simulink model "gtm_aeromodel"  (Simulink 7.2)
settings: Solver=ode45  StartTime=0.0  StopTime=10.0  RelTol=1e-3
undefined symbols (not defined in the file or in its folder): A_BLCG, A_BW, A_CW, A_FSCG, A_FSREF_in, A_SW, A_WLCG, A_WLREF, ALPHA0, bclowb, bclowbx_FMACH, bcmowb, bcmowbx_FHP, bcmowby_FMACH, cda, cdax_FLPDEF, cddr, cddrx_FMACH, cdo, cdox_FLPDEF, cdt1, cdt1x_mach, cdt2, cdt2x_mach, cdto, cdtox_mach, cdwb, cdwbx_FALPHA, cdwby_FMACH, clat, clatfr, clatfrx_FHP, clatfry_FMACH, clatx_mach, clawbfr, clawbfrx_FHP, clawbfry_FMACH, cldefr, cldefrx_FHP, cldefry_FMACH, cldtab, cldtabx_FMACH, clqwb, clqwbfr, clqwbfrx_FHP, clqwbfry_FMACH, clqwbx_mach, cltdd, cltddx_FHP, cltddy_FMACH, clwb, clwbtdd, clwbtddx_FHP, clwbtddy_FMACH, clwbx_FALPHA, clwby_FMACH, clwbzdd, clwbzddx_FHP, clwbzddy_FMACH, clzdd ... (+196)
libraries: model_lib x1
(part 1 of 10)
settings Model: Creator=E183308  LastModifiedBy=E183308

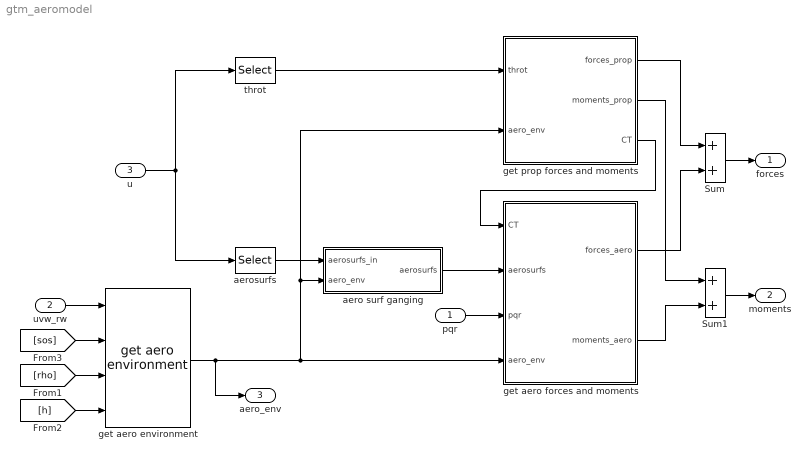
== system gtm_aeromodel ==
  pqr : Inport  OutDataType=sfix(16)  OutScaling=2^0
  uvw_rw : Inport  Port=2  OutDataType=sfix(16)  OutScaling=2^0
  u : Inport  Port=3  OutDataType=sfix(16)  OutScaling=2^0
  Sum : Sum  OutDataType=sfix(16)  OutScaling=2^0
  Sum1 : Sum  OutDataType=sfix(16)  OutScaling=2^0
  aero surf ganging : Subsystem
  aerosurfs : Selector  InputPortWidth=num_u  IndexOptions=Index vector (dialog)  Indices=vane_idx  OutputSizes=1
  get aero environment : model_lib/get aero environment  SystemSampleTime=-1
  get aero forces and moments : Subsystem
  get prop forces and moments : Subsystem
  throt : Selector  InputPortWidth=num_u  IndexOptions=Index vector (dialog)  Indices=throttle_idx  OutputSizes=1
  forces : Outport  OutDataType=sfix(16)  OutScaling=2^0
  moments : Outport  Port=2  OutDataType=sfix(16)  OutScaling=2^0
  aero_env : Outport  Port=3  OutDataType=sfix(16)  OutScaling=2^0
  wires:
  [h] -> get aero environment/4
  [sos] -> get aero environment/2
  [rho] -> get aero environment/3
  u/1 -> aerosurfs/1, throt/1
  uvw_rw/1 -> get aero environment/1
  throt/1 -> get prop forces and moments/1(throt)
  aerosurfs/1 -> aero surf ganging/1(aerosurfs_in)
  Sum/1 -> forces/1
  Sum1/1 -> moments/1
  get prop forces and moments/1(forces_prop) -> Sum/1
  get aero forces and moments/1(forces_aero) -> Sum/2
  get prop forces and moments/2(moments_prop) -> Sum1/1
  get prop forces and moments/3(CT) -> get aero forces and moments/1(CT)
  get aero forces and moments/2(moments_aero) -> Sum1/2
  pqr/1 -> get aero forces and moments/3(pqr)
  aero surf ganging/1(aerosurfs) -> get aero forces and moments/2(aerosurfs)
  get aero environment/1 -> get aero forces and moments/4(aero_env), aero surf ganging/2(aero_env), get prop forces and moments/2(aero_env), aero_env/1

== system gtm_aeromodel/aero surf ganging ==
  aerosurfs_in : Inport  OutDataType=sfix(16)  OutScaling=2^0
  aero_env : Inport  Port=2  OutDataType=sfix(16)  OutScaling=2^0
  Bus Creator : BusCreator  Inputs=13
  Bus Selector1 : BusSelector  OutputSignals=qbar
  Constant : Constant  Value=0  OutDataType=sfix(16)  OutScaling=2^0
  Constant1 : Constant  Value=0  OutDataType=sfix(16)  OutScaling=2^0
  Demux : Demux  Outputs=7
  FLAP/DSTAB : Lookup  InputValues=dstabx_FLPDEF  Table=dstab  OutDataType=sfix(16)  OutScaling=2^0  SaturateOnIntegerOverflow=on
  Gain : Gain  Gain=-1  ParameterDataType=sfix(16)  ParameterScaling=2^0  OutDataType=sfix(16)  OutScaling=2^0
  Gain{1..4} (4 alike) : Gain  ParameterDataType=sfix(16)  ParameterScaling=2^0  OutDataType=sfix(16)  OutScaling=2^0
  SPOILER : Subsystem
  aerosurfs : Outport  OutDataType=sfix(16)  OutScaling=2^0
  wires:
  Constant1/1 -> Bus Creator/6  "flgail"
  Constant/1 -> Bus Creator/8  "atab"
  Gain1/1 -> Bus Creator/11  "dsb"
  Gain4/1 -> Bus Creator/7  "ailr"
  Gain3/1 -> Bus Creator/13  "dsr"
  Gain2/1 -> Bus Creator/12  "dsl"
  Demux/5 -> SPOILER/3(splr)  "stab"
  SPOILER/3(dsr) -> Gain3/1  "dsr"
  SPOILER/2(dsl) -> Gain2/1  "dsl"
  SPOILER/1(dsb) -> Gain1/1  "dsb"
  Bus Selector1/1 -> SPOILER/2(Qdyn)
  aero_env/1 -> Bus Selector1/1
  FLAP/DSTAB/1 -> Bus Creator/5  "stab"
  Demux/6 -> FLAP/DSTAB/1, Bus Creator/9  "flap"
  Demux/1 -> SPOILER/1(halfdail), Gain4/1, Gain/1  "ail"
  Bus Creator/1 -> aerosurfs/1
  aerosurfs_in/1 -> Demux/1
  Demux/7 -> Bus Creator/10  "gear"
  Demux/4 -> Bus Creator/4  "eltab"
  Demux/3 -> Bus Creator/3  "rud"
  Gain/1 -> Bus Creator/2  "aill"
  Demux/2 -> Bus Creator/1  "elev"

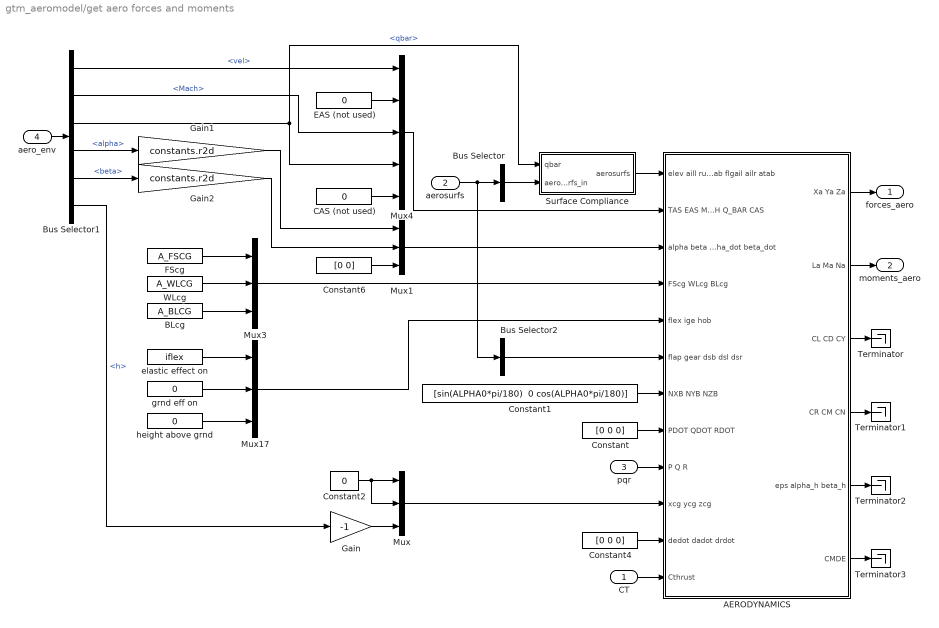
== system gtm_aeromodel/get aero forces and moments ==
  CT : Inport  OutDataType=sfix(16)  OutScaling=2^0
  aerosurfs : Inport  Port=2  OutDataType=sfix(16)  OutScaling=2^0
  pqr : Inport  Port=3  OutDataType=sfix(16)  OutScaling=2^0
  aero_env : Inport  Port=4  OutDataType=sfix(16)  OutScaling=2^0
  AERODYNAMICS : Subsystem
  BLcg : Constant  Value=A_BLCG  OutDataType=sfix(16)  OutScaling=2^0
  Bus Selector : BusSelector  OutputSignals=elev,aill,rud,eltab,stab,flgail,ailr,atab  OutputAsBus=on
  Bus Selector1 : BusSelector  OutputSignals=vel,Mach,qbar,alpha,beta,h
  Bus Selector2 : BusSelector  OutputSignals=flap,gear,dsb,dsl,dsr  OutputAsBus=on
  CAS (not used) : Constant  Value=0  OutDataType=sfix(16)  OutScaling=2^0
  Constant : Constant  Value=[0 0 0]  OutDataType=sfix(16)  OutScaling=2^0
  Constant1 : Constant  Value="[sin(ALPHA0*pi/180)  0 cos(ALPHA0*pi/180)]"  OutDataType=sfix(16)  OutScaling=2^0
  Constant2 : Constant  Value=0  OutDataType=sfix(16)  OutScaling=2^0
  Constant4 : Constant  Value=[0 0 0]  OutDataType=sfix(16)  OutScaling=2^0
  Constant6 : Constant  Value=[0 0]  OutDataType=sfix(16)  OutScaling=2^0
  EAS (not used) : Constant  Value=0  OutDataType=sfix(16)  OutScaling=2^0
  FScg : Constant  Value=A_FSCG  OutDataType=sfix(16)  OutScaling=2^0
  Gain : Gain  Gain=-1  ParameterDataType=sfix(16)  ParameterScaling=2^0  OutDataType=sfix(16)  OutScaling=2^0
  Gain1 : Gain  Gain=constants.r2d  ParameterDataType=sfix(16)  ParameterScaling=2^0  OutDataType=sfix(16)  OutScaling=2^0
  Gain2 : Gain  Gain=constants.r2d  ParameterDataType=sfix(16)  ParameterScaling=2^0  OutDataType=sfix(16)  OutScaling=2^0
  Mux : Mux  Inputs=3
  Mux1 : Mux  Inputs=[1 1 2]
  Mux17 : Mux  Inputs=3
  Mux3 : Mux  Inputs=3
  Mux4 : Mux  Inputs=5
  Surface Compliance : Subsystem
  Terminator{,1..3} (4 alike) : Terminator
  WLcg : Constant  Value=A_WLCG  OutDataType=sfix(16)  OutScaling=2^0
  elastic effect on : Constant  Value=iflex  OutDataType=sfix(16)  OutScaling=2^0
  grnd eff on : Constant  Value=0  OutDataType=sfix(16)  OutScaling=2^0
  height above grnd : Constant  Value=0  OutDataType=sfix(16)  OutScaling=2^0
  forces_aero : Outport  OutDataType=sfix(16)  OutScaling=2^0
  moments_aero : Outport  Port=2  OutDataType=sfix(16)  OutScaling=2^0
  wires:
  AERODYNAMICS/6(CMDE) -> Terminator3/1
  AERODYNAMICS/5(eps alpha_h beta_h) -> Terminator2/1
  AERODYNAMICS/4(CR CM CN) -> Terminator1/1
  AERODYNAMICS/3(CL CD CY) -> Terminator/1
  AERODYNAMICS/2(La Ma Na) -> moments_aero/1
  AERODYNAMICS/1("Xa Ya Za ") -> forces_aero/1
  Gain2/1 -> Mux1/2
  Gain1/1 -> Mux1/1
  Constant/1 -> AERODYNAMICS/8(PDOT QDOT RDOT)
  Constant1/1 -> AERODYNAMICS/7(NXB NYB NZB)
  pqr/1 -> AERODYNAMICS/9(P Q R)
  elastic effect on/1 -> Mux17/1
  grnd eff on/1 -> Mux17/2
  height above grnd/1 -> Mux17/3
  Bus Selector1/4 -> Gain1/1  "<alpha>"
  Mux1/1 -> AERODYNAMICS/3(alpha beta alpha_dot beta_dot)
  FScg/1 -> Mux3/1
  WLcg/1 -> Mux3/2
  BLcg/1 -> Mux3/3
  Mux3/1 -> AERODYNAMICS/4(FScg WLcg BLcg)
  Mux17/1 -> AERODYNAMICS/5(flex ige hob)
  EAS (not used)/1 -> Mux4/2
  Bus Selector1/3 -> Mux4/4, Surface Compliance/1(qbar)  "<qbar>"
  CAS (not used)/1 -> Mux4/5
  Bus Selector1/2 -> Mux4/3  "<Mach>"
  Mux4/1 -> AERODYNAMICS/2(TAS EAS MACH Q_BAR CAS)
  Constant6/1 -> Mux1/3
  Bus Selector1/5 -> Gain2/1  "<beta>"
  Bus Selector1/1 -> Mux4/1  "<vel>"
  aero_env/1 -> Bus Selector1/1
  Mux/1 -> AERODYNAMICS/10(xcg ycg zcg)
  Constant4/1 -> AERODYNAMICS/11(dedot dadot drdot)
  CT/1 -> AERODYNAMICS/12(Cthrust)
  Constant2/1 -> Mux/1, Mux/2
  Gain/1 -> Mux/3
  Bus Selector1/6 -> Gain/1  "<h>"
  aerosurfs/1 -> Bus Selector/1, Bus Selector2/1
  Bus Selector/1 -> Surface Compliance/2(aerosurfs_in)
  Bus Selector2/1 -> AERODYNAMICS/6(flap gear dsb dsl dsr)
  Surface Compliance/1(aerosurfs) -> AERODYNAMICS/1(elev aill rud eltab stab flgail ailr atab)

== system gtm_aeromodel/get prop forces and moments ==
  throt : Inport  OutDataType=sfix(16)  OutScaling=2^0
  aero_env : Inport  Port=2  OutDataType=sfix(16)  OutScaling=2^0
  Bus Selector : BusSelector  OutputSignals=qbar,Mach,h
  Constant1 : Constant  Value=4  VectorParams1D=off  OutDataType=sfix(16)  OutScaling=2^0
  Constant2 : Constant  Value=A_WLCG  VectorParams1D=off  OutDataType=sfix(16)  OutScaling=2^0
  ENGINE : Subsystem
  Engine inlet area (ft^2) : Constant  Value=12.57  VectorParams1D=off  OutDataType=sfix(16)  OutScaling=2^0
  Product3 : Product  Inputs=3  OutDataType=sfix(16)  OutScaling=2^0  RndMeth=Zero
  Terminator : Terminator
  Terminator1 : Terminator
  Terminator2 : Terminator
  forces_prop : Outport  OutDataType=sfix(16)  OutScaling=2^0
  moments_prop : Outport  Port=2  OutDataType=sfix(16)  OutScaling=2^0
  CT : Outport  Port=3  OutDataType=sfix(16)  OutScaling=2^0
  wires:
  throt/1 -> ENGINE/1(Thrust_Lever)
  ENGINE/1(Forces Prop) -> forces_prop/1
  ENGINE/2(Moments Prop) -> moments_prop/1
  ENGINE/3(CT) -> CT/1
  ENGINE/4(maxThrust) -> Terminator/1
  ENGINE/5(minThrust) -> Terminator1/1
  ENGINE/6(TRA) -> Terminator2/1
  Constant1/1 -> Product3/1
  Engine inlet area (ft^2)/1 -> Product3/2
  Product3/1 -> ENGINE/2(RamDrag0)
  Constant2/1 -> ENGINE/6(A_WLCG)
  aero_env/1 -> Bus Selector/1
  Bus Selector/1 -> Product3/3, ENGINE/3(Q_Bar0)  "<qbar>"
  Bus Selector/2 -> ENGINE/4(Mach)  "<Mach>"
  Bus Selector/3 -> ENGINE/5(Alt)  "<h>"

== system gtm_aeromodel/aero surf ganging/SPOILER ==
  note: isp
  halfdail : Inport  OutDataType=sfix(16)  OutScaling=2^0
  Qdyn : Inport  Port=2  OutDataType=sfix(16)  OutScaling=2^0
  splr : Inport  Port=3  OutDataType=sfix(16)  OutScaling=2^0
  Gain3 : Gain  Gain=-1  ParameterDataType=sfix(16)  ParameterScaling=2^0  OutDataType=sfix(16)  OutScaling=2^0  SaturateOnIntegerOverflow=on  OutDataTypeStr=Inherit: Same as input  ParamDataTypeStr=Inherit: Same as input
  Model Info : Subsystem  LoadFcn=slcm LoadBlock;  InitFcn=slcm('UpdateAllCMBlocksInThisModelInit')  mask(CMBlock){InitialSaveTempField=, InitialBlockCM=None, BlockCM=none, Frame=on, SaveTempField=, DisplayStringWithTags=|, MaskDisplayString=Model Name: SPOILER   Rev.: -\nDescription: Spoiler\nProgram: Planeview GV \nNext Block: ACTUATORS\nWritten by: G. Chan     Date: 06/28/00, HorizontalTextAlignment=Left, LeftAlignmentValue=0.02, SourceBlockDiagram=models, TagMaxNumber=20, CMTag1=, CMTag2=, CMTag3=, CMTag4=, CMTag5=, CMTag6=, CMTag7=, CMTag8=, CMTag9=, CMTag10=, CMTag11=, CMTag12=, CMTag13=, CMTag14=, CMTag15=, CMTag16=, CMTag17=, CMTag18=, CMTag19=, CMTag20=}
      mask DisplayStringWithTags=|
      | Model Name: SPOILER   Rev.: -
      | Description: Spoiler
      | Program: Planeview GV
      | Next Block: ACTUATORS
      | Written by: G. Chan     Date: 06/28/00
      mask help: This block allows revision control information to be displayed within the model.
      settings: CopyFcn=slcm CopyBlock;  DeleteFcn=slcm Cancel;  PostSaveFcn=slcm('UpdateAllCMBlocksInThisModel')  NameChangeFcn=slcm Rename;  OpenFcn=slcm
      mask Display: text(str2num(LeftAlignmentValue), 0.5, MaskDisplayString, 'HorizontalAlignment', HorizontalTextAlignment)
  Saturation : Saturate  UpperLimit=70  LowerLimit=0
  Saturation1 : Saturate  UpperLimit=70  LowerLimit=0
  Switch : Switch  Threshold=.5  SaturateOnIntegerOverflow=on  InputSameDT=on
  Switch1 : Switch  Threshold=.5  SaturateOnIntegerOverflow=on  InputSameDT=on
  dsl_ : Constant  Value=0  OutDataType=sfix(16)  OutScaling=2^0
  dsl_1 : Sum  OutDataType=sfix(16)  OutScaling=2^0  SaturateOnIntegerOverflow=on  InputSameDT=on  OutDataTypeStr=Inherit: Same as first input
  dslgear_1 : Subsystem  mask(2-D Table){y=dslgearx_FQ, z=dslgeary_DAILL, tab=dslgear}
      mask prompts: y "Y vector:"; z "Z vector:"; tab "Table:"
      mask help: 2-D Table Look Up. Enter monotonic Y and Z vectors and a matrix of 2-D tables. See the help for more info.
      mask Help: The Y and Z vectors must be monotonic.  Y  indexes into the columns of the 2-D table & Z indexes into the rows of the 2-D tables.   The input values are y and z respectively (e.g., top port = y).
      mask Display: plot(-10,-10,110,110,[90,50,10],[90,40,30],[90,50,10],[50,26,20],[90,50,10],[22,13,10])
  dsr_ : Constant  Value=0  OutDataType=sfix(16)  OutScaling=2^0
  dsr_1 : Sum  OutDataType=sfix(16)  OutScaling=2^0  SaturateOnIntegerOverflow=on  InputSameDT=on  OutDataTypeStr=Inherit: Same as first input
  dsrgear_ : Subsystem  mask(2-D Table){y=dsrgearx_FQ, z=dsrgeary_DAILR, tab=dsrgear}
      mask prompts: y "Y vector:"; z "Z vector:"; tab "Table:"
      mask help: 2-D Table Look Up. Enter monotonic Y and Z vectors and a matrix of 2-D tables. See the help for more info.
      mask Help: The Y and Z vectors must be monotonic.  Y  indexes into the columns of the 2-D table & Z indexes into the rows of the 2-D tables.   The input values are y and z respectively (e.g., top port = y).
      mask Display: plot(-10,-10,110,110,[90,50,10],[90,40,30],[90,50,10],[50,26,20],[90,50,10],[22,13,10])
  gearStatus3 : Constant  OutDataType=sfix(16)  OutScaling=2^0
  dsb : Outport  OutDataType=sfix(16)  OutScaling=2^0
  dsl : Outport  Port=2  OutDataType=sfix(16)  OutScaling=2^0
  dsr : Outport  Port=3  OutDataType=sfix(16)  OutScaling=2^0
  wires:
  halfdail/1 -> dsrgear_/2(Z), Gain3/1
  Qdyn/1 -> dslgear_1/1(Y), dsrgear_/1(Y)
  Gain3/1 -> dslgear_1/2(Z)
  dslgear_1/1(Interp Value) -> Switch/1
  dsrgear_/1(Interp Value) -> Switch1/1
  Saturation1/1 -> dsr/1
  dsr_1/1 -> Saturation1/1
  Saturation/1 -> dsl/1
  dsl_1/1 -> Saturation/1
  dsr_/1 -> Switch1/3
  dsl_/1 -> Switch/3
  Switch1/1 -> dsr_1/2
  gearStatus3/1 -> Switch1/2, Switch/2
  Switch/1 -> dsl_1/2
  splr/1 -> dsr_1/1, dsl_1/1, dsb/1

== system gtm_aeromodel/get aero forces and moments/AERODYNAMICS ==
  elev aill rud eltab stab flgail ailr atab : Inport  OutDataType=sfix(16)  OutScaling=2^0
  TAS EAS MACH Q_BAR CAS : Inport  Port=2  OutDataType=sfix(16)  OutScaling=2^0
  alpha beta alpha_dot beta_dot : Inport  Port=3  OutDataType=sfix(16)  OutScaling=2^0
  FScg WLcg BLcg : Inport  Port=4  OutDataType=sfix(16)  OutScaling=2^0
  flex ige hob : Inport  Port=5  OutDataType=sfix(16)  OutScaling=2^0
  flap gear dsb dsl dsr : Inport  Port=6  OutDataType=sfix(16)  OutScaling=2^0
  NXB NYB NZB : Inport  Port=7  OutDataType=sfix(16)  OutScaling=2^0
  PDOT QDOT RDOT : Inport  Port=8  OutDataType=sfix(16)  OutScaling=2^0
  P Q R : Inport  Port=9  OutDataType=sfix(16)  OutScaling=2^0
  xcg ycg zcg : Inport  Port=10  OutDataType=sfix(16)  OutScaling=2^0
  dedot dadot drdot : Inport  Port=11  OutDataType=sfix(16)  OutScaling=2^0
  Cthrust : Inport  Port=12  OutDataType=sfix(16)  OutScaling=2^0
  Aero Incidence Angles : Subsystem
  Force  Coefficients : Subsystem
  Moment Coefficients : Subsystem
  Mux : Mux  Inputs=3
  NONDIMRATE : Subsystem
  XFORMATION of  AERO FORCES and MOMENTS   to cg centered body axis : Subsystem
  sin2 : Fcn  Expr=-u[3]
  "Xa Ya Za " : Outport  OutDataType=sfix(16)  OutScaling=2^0  InitialOutput=0
  La Ma Na : Outport  Port=2  OutDataType=sfix(16)  OutScaling=2^0  InitialOutput=0
  CL CD CY : Outport  Port=3  OutDataType=sfix(16)  OutScaling=2^0  InitialOutput=0
  CR CM CN : Outport  Port=4  OutDataType=sfix(16)  OutScaling=2^0  InitialOutput=0
  eps alpha_h beta_h : Outport  Port=5  OutDataType=sfix(16)  OutScaling=2^0  InitialOutput=0
  CMDE : Outport  Port=6  OutDataType=sfix(16)  OutScaling=2^0  InitialOutput=0
  wires:
  Moment Coefficients/2(CMDE) -> CMDE/1
  NXB NYB NZB/1 -> Aero Incidence Angles/6(NXB NYB NZB), Moment Coefficients/9(NXB NYB NZB), Force  Coefficients/10(NXB NYB NZB)
  sin2/1 -> Aero Incidence Angles/2(alt), Moment Coefficients/7(alt), Force  Coefficients/8(alt)
  xcg ycg zcg/1 -> sin2/1
  Mux/1 -> eps alpha_h beta_h/1
  Aero Incidence Angles/3(betat) -> Mux/3, Force  Coefficients/12(beta_h), Moment Coefficients/12(beta_h)
  Aero Incidence Angles/1(eps) -> Mux/1, Force  Coefficients/2(eps)
  Aero Incidence Angles/2(alphat) -> Mux/2, Force  Coefficients/6(alpha_h), Moment Coefficients/5(alpha_h)
  Cthrust/1 -> Aero Incidence Angles/7(cthrust)
  PDOT QDOT RDOT/1 -> Force  Coefficients/11(PDOT QDOT RDOT), Moment Coefficients/10(PDOT QDOT RDOT)
  alpha beta alpha_dot beta_dot/1 -> Aero Incidence Angles/9(alpha beta alpha_dot beta_dot), NONDIMRATE/2(alpha beta eps_h alpha_h), Force  Coefficients/3(alpha beta alpha_dot beta_dot), Moment Coefficients/2(alpha beta alpha_dot beta_dot), XFORMATION of  AERO FORCES and MOMENTS   to cg centered body axis/3(alpha beta alpha_dot beta_dot)
  P Q R/1 -> Aero Incidence Angles/8(P Q R), NONDIMRATE/1(P Q R)
  TAS EAS MACH Q_BAR CAS/1 -> XFORMATION of  AERO FORCES and MOMENTS   to cg centered body axis/1(Vtas EASkts Mach Qdyn CASkts), Aero Incidence Angles/1(TAS EAS MACH Q_BAR CAS), NONDIMRATE/3(Vtas EASkts Mach Qdyn CASkts), Force  Coefficients/4(TAS EAS MACH Q_BAR CAS), Moment Coefficients/3(TAS EAS MACH Q_BAR CAS)
  XFORMATION of  AERO FORCES and MOMENTS   to cg centered body axis/2(La Ma Na) -> La Ma Na/1
  XFORMATION of  AERO FORCES and MOMENTS   to cg centered body axis/1(Xa Ya Za) -> "Xa Ya Za "/1
  dedot dadot drdot/1 -> Moment Coefficients/11(dedot dadot drdot)
  FScg WLcg BLcg/1 -> XFORMATION of  AERO FORCES and MOMENTS   to cg centered body axis/5(FScg WLcg BLcg)
  NONDIMRATE/1(P' Q' R') -> Force  Coefficients/5(P' Q' R'), Moment Coefficients/4(PHAT QHAT RHAT)
  flex ige hob/1 -> Aero Incidence Angles/3(flex ige hob), Moment Coefficients/1(flex ige hob), Force  Coefficients/1("flex ige hob ")
  elev aill rud eltab stab flgail ailr atab/1 -> Aero Incidence Angles/5(ctrl_surfaces), Moment Coefficients/6(elev aill rud eltab stab flgail ailr atab), Force  Coefficients/7(elev aill rud eltab stab flgail ailr atab)
  flap gear dsb dsl dsr/1 -> Aero Incidence Angles/4(flap gear dsb dsl dsr), Moment Coefficients/8(flap gear dsb dsl dsr), Force  Coefficients/9(flap gear dsb dsl dsr)
  Force  Coefficients/1(CL CD CY) -> XFORMATION of  AERO FORCES and MOMENTS   to cg centered body axis/2(CL CD CY), CL CD CY/1
  Moment Coefficients/1(CR CM CN) -> XFORMATION of  AERO FORCES and MOMENTS   to cg centered body axis/4(CR CM CN), CR CM CN/1

== system gtm_aeromodel/get aero forces and moments/Surface Compliance ==
  qbar : Inport  OutDataType=sfix(16)  OutScaling=2^0
  aerosurfs_in : Inport  Port=2  OutDataType=sfix(16)  OutScaling=2^0
  Aileron Compliance : Lookup  InputValues="[0  92  221]"  Table="[1  0.85  0.8]"  OutDataType=sfix(16)  OutScaling=2^0  SaturateOnIntegerOverflow=on
  Demux : Demux  Outputs=[1 1 6]
  Elevator Compliance : Lookup  InputValues=[0 46 132 200 300 400]  Table="[1   1  0.7  0.65 0.6 0.4]"  OutDataType=sfix(16)  OutScaling=2^0  SaturateOnIntegerOverflow=on
  Mux : Mux  Inputs=3
  Product : Product  OutDataType=sfix(16)  OutScaling=2^0  RndMeth=Zero
  Product1 : Product  OutDataType=sfix(16)  OutScaling=2^0  RndMeth=Zero
  aerosurfs : Outport  OutDataType=sfix(16)  OutScaling=2^0
  wires:
  Mux/1 -> aerosurfs/1
  Demux/1 -> Product/2
  Demux/2 -> Product1/2
  Product/1 -> Mux/1
  aerosurfs_in/1 -> Demux/1
  Demux/3 -> Mux/3
  Elevator Compliance/1 -> Product/1
  qbar/1 -> Aileron Compliance/1, Elevator Compliance/1
  Product1/1 -> Mux/2
  Aileron Compliance/1 -> Product1/1

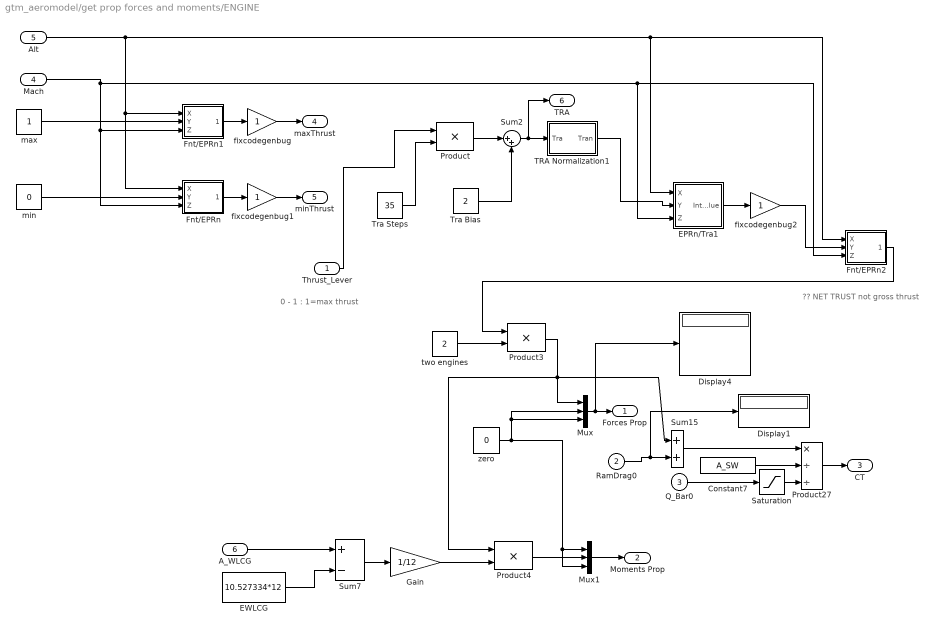
== system gtm_aeromodel/get prop forces and moments/ENGINE ==
  note: ?? NET TRUST not gross thrust
  note: 0 - 1 : 1=max thrust
  Thrust_Lever : Inport  OutDataType=sfix(16)  OutScaling=2^0
  RamDrag0 : Inport  Port=2  OutDataType=sfix(16)  OutScaling=2^0
  Q_Bar0 : Inport  Port=3  OutDataType=sfix(16)  OutScaling=2^0
  Mach : Inport  Port=4  OutDataType=sfix(16)  OutScaling=2^0
  Alt : Inport  Port=5  OutDataType=sfix(16)  OutScaling=2^0
  A_WLCG : Inport  Port=6  OutDataType=sfix(16)  OutScaling=2^0
  Constant7 : Constant  Value=A_SW  OutDataType=sfix(16)  OutScaling=2^0
  Display1 : Display
  Display4 : Display
  EPRn/Tra1 : Subsystem  mask(1-2-3 Table){@1=altvec, @2=sstravec, @3=machvec, @4=eprn_tra}
      mask prompts: @1 "X vector:"; @2 "Y vector:"; @3 "Z vector:"; @4 "Table:"
      mask help: 3-D Table Look Up. Enter monotonic X, Y and Z vectors and a matrix of 2-D tables. See the help for more info.
      mask init:
      | x=@1;y=@2;z=@3;tab=@4;
      mask Help: The X, Y and Z vectors must be monotonic.   The 3-D table is a horizontal concatenation of  2-D tables.  X  indexes into the columns of the 2-D tables & Y indexes into the rows of the 2-D tables.  Z indexes into the table levels (starting with the 1st 2-D table).   The input values are x, y and z respectively (e.g., top port = x).
      mask Display: plot([0 2 2 0 0],[0 0 2 2 0],[0 2 2.9 0.95 0],[2 2 2.7 2.7 2],[2 2.9 2.9 2 2],[0 0.85 2.7 2 0])
  EWLCG : Constant  Value=10.527334*12  OutDataType=sfix(16)  OutScaling=2^0
  Fnt/EPRn : Subsystem  mask(1-2-3 Table){@1=altvec, @2=sseprvec, @3=machvec, @4=fn_epr}
      mask prompts: @1 "X vector:"; @2 "Y vector:"; @3 "Z vector:"; @4 "Table:"
      mask help: 3-D Table Look Up. Enter monotonic X, Y and Z vectors and a matrix of 2-D tables. See the help for more info.
      mask init:
      | x=@1;y=@2;z=@3;tab=@4;
      mask Help: The X, Y and Z vectors must be monotonic.   The 3-D table is a horizontal concatenation of  2-D tables.  X  indexes into the columns of the 2-D tables & Y indexes into the rows of the 2-D tables.  Z indexes into the table levels (starting with the 1st 2-D table).   The input values are x, y and z respectively (e.g., top port = x).
      mask Display: plot([0 2 2 0 0],[0 0 2 2 0],[0 2 2.9 0.95 0],[2 2 2.7 2.7 2],[2 2.9 2.9 2 2],[0 0.85 2.7 2 0])
  Fnt/EPRn1 : Subsystem  mask(1-2-3 Table){@1=altvec, @2=sseprvec, @3=machvec, @4=fn_epr}
      mask prompts: @1 "X vector:"; @2 "Y vector:"; @3 "Z vector:"; @4 "Table:"
      mask help: 3-D Table Look Up. Enter monotonic X, Y and Z vectors and a matrix of 2-D tables. See the help for more info.
      mask init:
      | x=@1;y=@2;z=@3;tab=@4;
      mask Help: The X, Y and Z vectors must be monotonic.   The 3-D table is a horizontal concatenation of  2-D tables.  X  indexes into the columns of the 2-D tables & Y indexes into the rows of the 2-D tables.  Z indexes into the table levels (starting with the 1st 2-D table).   The input values are x, y and z respectively (e.g., top port = x).
      mask Display: plot([0 2 2 0 0],[0 0 2 2 0],[0 2 2.9 0.95 0],[2 2 2.7 2.7 2],[2 2.9 2.9 2 2],[0 0.85 2.7 2 0])
  Fnt/EPRn2 : Subsystem  mask(1-2-3 Table){@1=altvec, @2=sseprvec, @3=machvec, @4=fn_epr}
      mask prompts: @1 "X vector:"; @2 "Y vector:"; @3 "Z vector:"; @4 "Table:"
      mask help: 3-D Table Look Up. Enter monotonic X, Y and Z vectors and a matrix of 2-D tables. See the help for more info.
      mask init:
      | x=@1;y=@2;z=@3;tab=@4;
      mask Help: The X, Y and Z vectors must be monotonic.   The 3-D table is a horizontal concatenation of  2-D tables.  X  indexes into the columns of the 2-D tables & Y indexes into the rows of the 2-D tables.  Z indexes into the table levels (starting with the 1st 2-D table).   The input values are x, y and z respectively (e.g., top port = x).
      mask Display: plot([0 2 2 0 0],[0 0 2 2 0],[0 2 2.9 0.95 0],[2 2 2.7 2.7 2],[2 2.9 2.9 2 2],[0 0.85 2.7 2 0])
  Gain : Gain  Gain=1/12  ParameterDataType=sfix(16)  ParameterScaling=2^0  OutDataType=sfix(16)  OutScaling=2^0  SaturateOnIntegerOverflow=on  OutDataTypeStr=Inherit: Same as input  ParamDataTypeStr=Inherit: Same as input
  Mux : Mux  Inputs=3
  Mux1 : Mux  Inputs=3
  Product : Product  OutDataType=sfix(16)  OutScaling=2^0  SaturateOnIntegerOverflow=on  RndMeth=Zero  InputSameDT=on  OutDataTypeStr=Inherit: Same as first input
  Product27 : Product  Inputs=*//  OutDataType=sfix(16)  OutScaling=2^0  SaturateOnIntegerOverflow=on  RndMeth=Zero  InputSameDT=on  OutDataTypeStr=Inherit: Same as first input
  Product3 : Product  OutDataType=sfix(16)  OutScaling=2^0  SaturateOnIntegerOverflow=on  RndMeth=Zero  InputSameDT=on  OutDataTypeStr=Inherit: Same as first input
  Product4 : Product  OutDataType=sfix(16)  OutScaling=2^0  SaturateOnIntegerOverflow=on  RndMeth=Zero  InputSameDT=on  OutDataTypeStr=Inherit: Same as first input
  Saturation : Saturate  UpperLimit=inf  LowerLimit=0.1
  Sum15 : Sum  OutDataType=sfix(16)  OutScaling=2^0  SaturateOnIntegerOverflow=on  InputSameDT=on  OutDataTypeStr=Inherit: Same as first input
  Sum2 : Sum  Inputs=|++  OutDataType=sfix(16)  OutScaling=2^0  SaturateOnIntegerOverflow=on  InputSameDT=on  OutDataTypeStr=Inherit: Same as first input
  Sum7 : Sum  Inputs=+-  OutDataType=sfix(16)  OutScaling=2^0  SaturateOnIntegerOverflow=on  InputSameDT=on  OutDataTypeStr=Inherit: Same as first input
  TRA Normalization1 : Subsystem
  Tra Bias : Constant  Value=2  OutDataType=sfix(16)  OutScaling=2^0
  Tra Steps : Constant  Value=35  OutDataType=sfix(16)  OutScaling=2^0
  fixcodegenbug : Gain  ParameterDataType=sfix(16)  ParameterScaling=2^0  OutDataType=sfix(16)  OutScaling=2^0  SaturateOnIntegerOverflow=on  OutDataTypeStr=Inherit: Same as input  ParamDataTypeStr=Inherit: Same as input
  fixcodegenbug1 : Gain  ParameterDataType=sfix(16)  ParameterScaling=2^0  OutDataType=sfix(16)  OutScaling=2^0  SaturateOnIntegerOverflow=on  OutDataTypeStr=Inherit: Same as input  ParamDataTypeStr=Inherit: Same as input
  fixcodegenbug2 : Gain  ParameterDataType=sfix(16)  ParameterScaling=2^0  OutDataType=sfix(16)  OutScaling=2^0  SaturateOnIntegerOverflow=on  OutDataTypeStr=Inherit: Same as input  ParamDataTypeStr=Inherit: Same as input
  max : Constant  OutDataType=sfix(16)  OutScaling=2^0
  min : Constant  Value=0  OutDataType=sfix(16)  OutScaling=2^0
  two engines : Constant  Value=2  OutDataType=sfix(16)  OutScaling=2^0
  zero : Constant  Value=0  OutDataType=sfix(16)  OutScaling=2^0
  Forces Prop : Outport  OutDataType=sfix(16)  OutScaling=2^0
  Moments Prop : Outport  Port=2  OutDataType=sfix(16)  OutScaling=2^0
  CT : Outport  Port=3  OutDataType=sfix(16)  OutScaling=2^0
  maxThrust : Outport  Port=4  OutDataType=sfix(16)  OutScaling=2^0
  minThrust : Outport  Port=5  OutDataType=sfix(16)  OutScaling=2^0
  TRA : Outport  Port=6  OutDataType=sfix(16)  OutScaling=2^0
  wires:
  Mach/1 -> Fnt/EPRn/3(Z), Fnt/EPRn1/3(Z), EPRn/Tra1/3(Z), Fnt/EPRn2/3(Z)
  Alt/1 -> Fnt/EPRn/1(X), Fnt/EPRn1/1(X), EPRn/Tra1/1(X), Fnt/EPRn2/1(X)
  max/1 -> Fnt/EPRn1/2(Y)
  min/1 -> Fnt/EPRn/2(Y)
  Fnt/EPRn/1(Interp Value) -> fixcodegenbug1/1
  Fnt/EPRn1/1(Interp Value) -> fixcodegenbug/1
  Tra Steps/1 -> Product/2
  Product/1 -> Sum2/1
  Tra Bias/1 -> Sum2/2
  TRA Normalization1/1(Tran) -> EPRn/Tra1/2(Y)
  EPRn/Tra1/1(Interp Value) -> fixcodegenbug2/1
  Fnt/EPRn2/1(Interp Value) -> Product3/1
  zero/1 -> Mux/2, Mux/3, Mux1/1, Mux1/3
  Product3/1 -> Mux/1, Product4/1, Sum15/1
  Mux/1 -> Forces Prop/1, Display4/1
  Sum7/1 -> Gain/1
  EWLCG/1 -> Sum7/2
  A_WLCG/1 -> Sum7/1
  two engines/1 -> Product3/2
  Product4/1 -> Mux1/2
  Mux1/1 -> Moments Prop/1
  Saturation/1 -> Product27/3
  Q_Bar0/1 -> Saturation/1
  Product27/1 -> CT/1
  Constant7/1 -> Product27/2
  Sum15/1 -> Product27/1
  RamDrag0/1 -> Sum15/2, Display1/1
  Sum2/1 -> TRA/1, TRA Normalization1/1(Tra)
  Gain/1 -> Product4/2
  Thrust_Lever/1 -> Product/1
  fixcodegenbug/1 -> maxThrust/1
  fixcodegenbug1/1 -> minThrust/1
  fixcodegenbug2/1 -> Fnt/EPRn2/2(Y)

== system gtm_aeromodel/aero surf ganging/SPOILER/Model Info ==
  EmptySubsystem : Subsystem

== system gtm_aeromodel/aero surf ganging/SPOILER/dslgear_1 ==
  Y : Inport  OutDataType=sfix(16)  OutScaling=2^0
  Z : Inport  Port=2  OutDataType=sfix(16)  OutScaling=2^0
  Mux : Mux  Inputs=2
  S-Function : S-Function  FunctionName=table2v5  Parameters=y,z,tab  EnableBusSupport=off
  Interp Value : Outport  OutDataType=sfix(16)  OutScaling=2^0
  wires:
  Z/1 -> Mux/2
  Y/1 -> Mux/1
  S-Function/1 -> Interp Value/1
  Mux/1 -> S-Function/1

== system gtm_aeromodel/aero surf ganging/SPOILER/dsrgear_ ==
  Y : Inport  OutDataType=sfix(16)  OutScaling=2^0
  Z : Inport  Port=2  OutDataType=sfix(16)  OutScaling=2^0
  Mux : Mux  Inputs=2
  S-Function : S-Function  FunctionName=table2v5  Parameters=y,z,tab  EnableBusSupport=off
  Interp Value : Outport  OutDataType=sfix(16)  OutScaling=2^0
  wires:
  Mux/1 -> S-Function/1
  S-Function/1 -> Interp Value/1
  Y/1 -> Mux/1
  Z/1 -> Mux/2

== system gtm_aeromodel/get aero forces and moments/AERODYNAMICS/Aero Incidence Angles ==
  TAS EAS MACH Q_BAR CAS : Inport  OutDataType=sfix(16)  OutScaling=2^0
  alt : Inport  Port=2  OutDataType=sfix(16)  OutScaling=2^0
  flex ige hob : Inport  Port=3  OutDataType=sfix(16)  OutScaling=2^0
  flap gear dsb dsl dsr : Inport  Port=4  OutDataType=sfix(16)  OutScaling=2^0
  ctrl_surfaces : Inport  Port=5  OutDataType=sfix(16)  OutScaling=2^0
  NXB NYB NZB : Inport  Port=6  OutDataType=sfix(16)  OutScaling=2^0
  cthrust : Inport  Port=7  OutDataType=sfix(16)  OutScaling=2^0
  P Q R : Inport  Port=8  OutDataType=sfix(16)  OutScaling=2^0
  alpha beta alpha_dot beta_dot : Inport  Port=9  OutDataType=sfix(16)  OutScaling=2^0
  DOWNWASH : Subsystem
  Fcn{,4,7,9,11} (5 alike) : Fcn  Expr=u[3]
  Fcn{1,3,5,8} (4 alike) : Fcn  Expr=u[1]
  Fcn10 : Fcn  Expr=u[4]
  Fcn12 : Fcn  Expr=u[2]*constants.g
  Fcn13 : Fcn  Expr=u[5]
  Fcn14 : Fcn  Expr=u[2]
  Fcn2 : Fcn  Expr=u[4]
  Fcn6 : Fcn  Expr=u[2]
  TAIL ANGLES : Subsystem
  beta : Fcn  Expr=u[2]
  elev : Fcn  Expr=u[1]
  eltab : Fcn  Expr=u[4]
  rud : Fcn  Expr=u[3]
  stab : Fcn  Expr=u[5]
  eps : Outport  OutDataType=sfix(16)  OutScaling=2^0
  alphat : Outport  Port=2  OutDataType=sfix(16)  OutScaling=2^0
  betat : Outport  Port=3  OutDataType=sfix(16)  OutScaling=2^0
  wires:
  alt/1 -> DOWNWASH/3(altitude), TAIL ANGLES/8(altitude)
  alpha beta alpha_dot beta_dot/1 -> beta/1, Fcn4/1, Fcn1/1
  ctrl_surfaces/1 -> rud/1, eltab/1, elev/1, stab/1
  Fcn12/1 -> TAIL ANGLES/13(side acc ft/s^2)
  Fcn11/1 -> TAIL ANGLES/5(NZB g's)
  Fcn10/1 -> DOWNWASH/9(dsl)
  Fcn9/1 -> DOWNWASH/8(dsb)
  TAS EAS MACH Q_BAR CAS/1 -> Fcn/1, Fcn2/1, Fcn3/1
  DOWNWASH/1(eps) -> TAIL ANGLES/3(eps), eps/1
  rud/1 -> TAIL ANGLES/12(rud)
  NXB NYB NZB/1 -> Fcn12/1, Fcn11/1
  TAIL ANGLES/2(betat) -> betat/1
  Fcn4/1 -> DOWNWASH/12(alphadot)
  Fcn1/1 -> DOWNWASH/1("alpha "), TAIL ANGLES/1(alpha)
  elev/1 -> TAIL ANGLES/6(elev)
  Fcn/1 -> DOWNWASH/2(mach), TAIL ANGLES/7(mach)
  Fcn2/1 -> DOWNWASH/10(qdyn), TAIL ANGLES/10(qdyn)
  eltab/1 -> TAIL ANGLES/9(el_tab)
  TAIL ANGLES/1(alphat) -> alphat/1
  flex ige hob/1 -> Fcn5/1, Fcn6/1, Fcn7/1
  Fcn7/1 -> DOWNWASH/6(hob)
  Fcn5/1 -> DOWNWASH/4(flex), TAIL ANGLES/4(flex)
  Fcn6/1 -> DOWNWASH/5(ige)
  Fcn8/1 -> DOWNWASH/7(flap)
  flap gear dsb dsl dsr/1 -> Fcn8/1, Fcn9/1, Fcn10/1, Fcn13/1
  stab/1 -> TAIL ANGLES/2(stab)
  Fcn13/1 -> DOWNWASH/13(dsr)
  cthrust/1 -> DOWNWASH/14(cthrust)
  DOWNWASH/2(xht) -> TAIL ANGLES/14(xht)
  P Q R/1 -> Fcn14/1
  Fcn3/1 -> DOWNWASH/11(TAS), TAIL ANGLES/16(TAS)
  beta/1 -> TAIL ANGLES/11(beta)
  Fcn14/1 -> TAIL ANGLES/15(q)

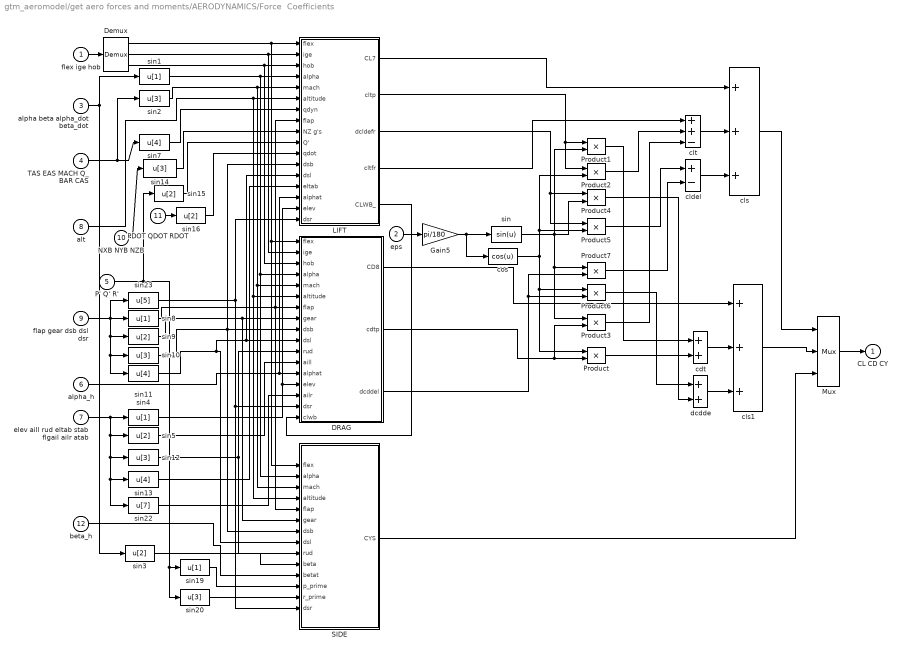
== system gtm_aeromodel/get aero forces and moments/AERODYNAMICS/Force  Coefficients ==
  "flex ige hob " : Inport  OutDataType=sfix(16)  OutScaling=2^0
  eps : Inport  Port=2  OutDataType=sfix(16)  OutScaling=2^0
  alpha beta alpha_dot beta_dot : Inport  Port=3  OutDataType=sfix(16)  OutScaling=2^0
  TAS EAS MACH Q_BAR CAS : Inport  Port=4  OutDataType=sfix(16)  OutScaling=2^0
  P' Q' R' : Inport  Port=5  OutDataType=sfix(16)  OutScaling=2^0
  alpha_h : Inport  Port=6  OutDataType=sfix(16)  OutScaling=2^0
  elev aill rud eltab stab flgail ailr atab : Inport  Port=7  OutDataType=sfix(16)  OutScaling=2^0
  alt : Inport  Port=8  OutDataType=sfix(16)  OutScaling=2^0
  flap gear dsb dsl dsr : Inport  Port=9  OutDataType=sfix(16)  OutScaling=2^0
  NXB NYB NZB : Inport  Port=10  OutDataType=sfix(16)  OutScaling=2^0
  PDOT QDOT RDOT : Inport  Port=11  OutDataType=sfix(16)  OutScaling=2^0
  beta_h : Inport  Port=12  OutDataType=sfix(16)  OutScaling=2^0
  "DRAG " : Subsystem
  Demux : Demux  Outputs=3
  Gain5 : Gain  Gain=pi/180  ParameterDataType=sfix(16)  ParameterScaling=2^0  OutDataType=sfix(16)  OutScaling=2^0  SaturateOnIntegerOverflow=on  OutDataTypeStr=Inherit: Same as input  ParamDataTypeStr=Inherit: Same as input
  LIFT : Subsystem
  Mux : Mux  Inputs=3
  Product{,1..7} (8 alike) : Product  OutDataType=sfix(16)  OutScaling=2^0  SaturateOnIntegerOverflow=on  RndMeth=Zero  InputSameDT=on  OutDataTypeStr=Inherit: Same as first input
  SIDE : Subsystem
  cdt : Sum  OutDataType=sfix(16)  OutScaling=2^0  SaturateOnIntegerOverflow=on  InputSameDT=on  OutDataTypeStr=Inherit: Same as first input
  cldel : Sum  Inputs=+-  OutDataType=sfix(16)  OutScaling=2^0  SaturateOnIntegerOverflow=on  InputSameDT=on  OutDataTypeStr=Inherit: Same as first input
  cls : Sum  Inputs=+++  OutDataType=sfix(16)  OutScaling=2^0  SaturateOnIntegerOverflow=on  InputSameDT=on  OutDataTypeStr=Inherit: Same as first input
  cls1 : Sum  Inputs=+++  OutDataType=sfix(16)  OutScaling=2^0  SaturateOnIntegerOverflow=on  InputSameDT=on  OutDataTypeStr=Inherit: Same as first input
  clt : Sum  Inputs=++-  OutDataType=sfix(16)  OutScaling=2^0  SaturateOnIntegerOverflow=on  InputSameDT=on  OutDataTypeStr=Inherit: Same as first input
  cos : Fcn  Expr=cos(u)
  dcdde : Sum  OutDataType=sfix(16)  OutScaling=2^0  SaturateOnIntegerOverflow=on  InputSameDT=on  OutDataTypeStr=Inherit: Same as first input
  sin : Fcn  Expr=sin(u)
  sin{1,4,8,19} (4 alike) : Fcn  Expr=u[1]
  sin{2,10,12,14,20} (5 alike) : Fcn  Expr=u[3]
  sin11 : Fcn  Expr=u[4]
  sin13 : Fcn  Expr=u[4]
  sin{3,5,9,15..16} (5 alike) : Fcn  Expr=u[2]
  sin22 : Fcn  Expr=u[7]
  sin23 : Fcn  Expr=u[5]
  sin7 : Fcn  Expr=u[4]
  CL CD CY : Outport  OutDataType=sfix(16)  OutScaling=2^0  InitialOutput=0
  wires:
  sin12/1 -> "DRAG "/11(rud), SIDE/9(rud)
  cls/1 -> Mux/1
  SIDE/1(CYS) -> Mux/3
  cls1/1 -> Mux/2
  cdt/1 -> cls1/2
  LIFT/1(CL7) -> cls/1
  cldel/1 -> cls/3
  clt/1 -> cls/2
  dcdde/1 -> cls1/3
  beta_h/1 -> SIDE/11(betat)
  alpha_h/1 -> "DRAG "/13(alphat), LIFT/15(alphat)
  sin4/1 -> "DRAG "/14(elev), LIFT/16(elev)
  alt/1 -> SIDE/4(altitude), "DRAG "/6(altitude), LIFT/6(altitude)
  sin22/1 -> "DRAG "/15(ailr)
  sin20/1 -> SIDE/13(r_prime)
  sin19/1 -> SIDE/12(p_prime)
  P' Q' R'/1 -> sin19/1, sin20/1, sin15/1
  sin10/1 -> LIFT/12(dsb), SIDE/7(dsb), "DRAG "/9(dsb)
  sin11/1 -> SIDE/8(dsl), "DRAG "/10(dsl), LIFT/13(dsl)
  sin3/1 -> SIDE/10(beta)
  "flex ige hob "/1 -> Demux/1
  Demux/2 -> LIFT/2(ige), "DRAG "/2(ige)
  Demux/1 -> "DRAG "/1(flex), SIDE/1(flex), LIFT/1(flex)
  LIFT/2(cltp) -> Product1/1, Product2/1
  "DRAG "/2(cdtp) -> Product/2, Product3/2
  LIFT/3(dcldefr) -> Product4/1, Product5/1
  "DRAG "/3(dcddel) -> Product6/2, Product7/2
  sin/1 -> Product3/1, Product7/1, Product1/2, Product4/2
  cos/1 -> Product6/1, Product/1, Product2/2, Product5/2
  Product/1 -> cdt/2
  Product6/1 -> dcdde/1
  Product7/1 -> cldel/2
  Product5/1 -> cldel/1
  Product4/1 -> dcdde/2
  LIFT/4(cltfr) -> clt/1
  Product3/1 -> clt/3
  Product2/1 -> clt/2
  Product1/1 -> cdt/1
  Gain5/1 -> cos/1, sin/1
  eps/1 -> Gain5/1
  Mux/1 -> CL CD CY/1
  Demux/3 -> "DRAG "/3(hob), LIFT/3(hob)
  sin1/1 -> "DRAG "/4(alpha), SIDE/2(alpha), LIFT/4(alpha)
  alpha beta alpha_dot beta_dot/1 -> sin1/1, sin3/1
  sin2/1 -> SIDE/3(mach), "DRAG "/5(mach), LIFT/5(mach)
  elev aill rud eltab stab flgail ailr atab/1 -> sin4/1, sin5/1, sin13/1, sin22/1, sin12/1
  sin5/1 -> "DRAG "/12(aill)
  TAS EAS MACH Q_BAR CAS/1 -> sin2/1, sin7/1
  sin7/1 -> LIFT/7(qdyn)
  flap gear dsb dsl dsr/1 -> sin8/1, sin9/1, sin10/1, sin11/1, sin23/1
  sin8/1 -> SIDE/5(flap), "DRAG "/7(flap), LIFT/8(flap)
  sin13/1 -> LIFT/14(eltab)
  sin9/1 -> SIDE/6(gear), "DRAG "/8(gear)
  NXB NYB NZB/1 -> sin14/1
  sin14/1 -> LIFT/9(NZ g's)
  sin15/1 -> LIFT/10(Q')
  sin16/1 -> LIFT/11(qdot)
  PDOT QDOT RDOT/1 -> sin16/1
  "DRAG "/1(CD8) -> cls1/1
  sin23/1 -> LIFT/17(dsr), "DRAG "/16(dsr), SIDE/14(dsr)
  LIFT/5(CLWB_) -> "DRAG "/17(clwb)

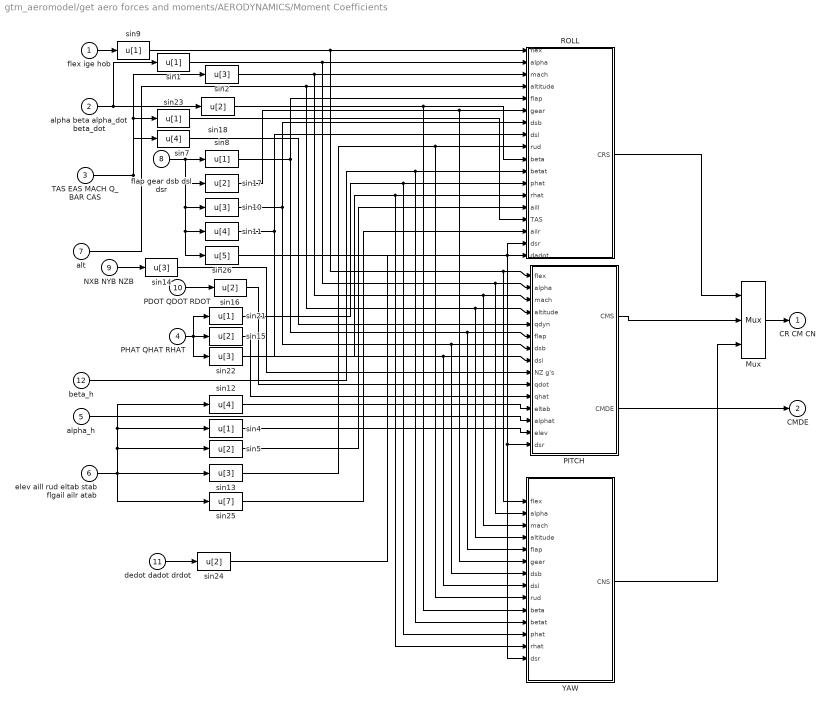
== system gtm_aeromodel/get aero forces and moments/AERODYNAMICS/Moment Coefficients ==
  flex ige hob : Inport  OutDataType=sfix(16)  OutScaling=2^0
  alpha beta alpha_dot beta_dot : Inport  Port=2  OutDataType=sfix(16)  OutScaling=2^0
  TAS EAS MACH Q_BAR CAS : Inport  Port=3  OutDataType=sfix(16)  OutScaling=2^0
  PHAT QHAT RHAT : Inport  Port=4  OutDataType=sfix(16)  OutScaling=2^0
  alpha_h : Inport  Port=5  OutDataType=sfix(16)  OutScaling=2^0
  elev aill rud eltab stab flgail ailr atab : Inport  Port=6  OutDataType=sfix(16)  OutScaling=2^0
  alt : Inport  Port=7  OutDataType=sfix(16)  OutScaling=2^0
  flap gear dsb dsl dsr : Inport  Port=8  OutDataType=sfix(16)  OutScaling=2^0
  NXB NYB NZB : Inport  Port=9  OutDataType=sfix(16)  OutScaling=2^0
  PDOT QDOT RDOT : Inport  Port=10  OutDataType=sfix(16)  OutScaling=2^0
  dedot dadot drdot : Inport  Port=11  OutDataType=sfix(16)  OutScaling=2^0
  beta_h : Inport  Port=12  OutDataType=sfix(16)  OutScaling=2^0
  Mux : Mux  Inputs=3
  PITCH : Subsystem
  ROLL : Subsystem
  YAW : Subsystem
  sin{1,4,8..9,21,23} (6 alike) : Fcn  Expr=u[1]
  sin{2,10,13..14,22} (5 alike) : Fcn  Expr=u[3]
  sin11 : Fcn  Expr=u[4]
  sin12 : Fcn  Expr=u[4]
  sin{5,15..18,24} (6 alike) : Fcn  Expr=u[2]
  sin25 : Fcn  Expr=u[7]
  sin26 : Fcn  Expr=u[5]
  sin7 : Fcn  Expr=u[4]
  CR CM CN : Outport  OutDataType=sfix(16)  OutScaling=2^0  InitialOutput=0
  CMDE : Outport  Port=2  OutDataType=sfix(16)  OutScaling=2^0  InitialOutput=0
  wires:
  PITCH/2(CMDE) -> CMDE/1
  YAW/1(CNS) -> Mux/3
  ROLL/1(CRS) -> Mux/1
  PITCH/1(CMS) -> Mux/2
  beta_h/1 -> YAW/11(betat), ROLL/11(betat)
  alpha_h/1 -> PITCH/13(alphat)
  alt/1 -> YAW/4(altitude), PITCH/4(altitude), ROLL/4(altitude)
  sin24/1 -> ROLL/18(dadot)
  dedot dadot drdot/1 -> sin24/1
  sin25/1 -> ROLL/16(ailr)
  elev aill rud eltab stab flgail ailr atab/1 -> sin13/1, sin25/1, sin12/1, sin5/1, sin4/1
  sin18/1 -> YAW/10(beta), ROLL/10(beta)
  sin13/1 -> YAW/9(rud), ROLL/9(rud)
  sin22/1 -> YAW/13(rhat), ROLL/13(rhat)
  sin21/1 -> YAW/12(phat), ROLL/12(phat)
  sin17/1 -> YAW/6(gear), ROLL/6(gear)
  sin23/1 -> ROLL/15(TAS)
  sin5/1 -> ROLL/14(aill)
  PHAT QHAT RHAT/1 -> sin22/1, sin21/1, sin15/1
  alpha beta alpha_dot beta_dot/1 -> sin18/1, sin1/1
  sin11/1 -> YAW/8(dsl), PITCH/8(dsl), ROLL/8(dsl)
  sin10/1 -> YAW/7(dsb), PITCH/7(dsb), ROLL/7(dsb)
  NXB NYB NZB/1 -> sin14/1
  PDOT QDOT RDOT/1 -> sin16/1
  sin8/1 -> YAW/5(flap), PITCH/6(flap), ROLL/5(flap)
  sin2/1 -> YAW/3(mach), PITCH/3(mach), ROLL/3(mach)
  sin1/1 -> YAW/2(alpha), PITCH/2(alpha), ROLL/2(alpha)
  sin9/1 -> YAW/1(flex), PITCH/1(flex), ROLL/1(flex)
  sin4/1 -> PITCH/14(elev)
  sin12/1 -> PITCH/12(eltab)
  flex ige hob/1 -> sin9/1
  TAS EAS MACH Q_BAR CAS/1 -> sin23/1, sin2/1, sin7/1
  sin7/1 -> PITCH/5(qdyn)
  flap gear dsb dsl dsr/1 -> sin17/1, sin10/1, sin11/1, sin26/1, sin8/1
  sin14/1 -> PITCH/9(NZ g's)
  sin16/1 -> PITCH/10(qdot)
  sin15/1 -> PITCH/11(qhat)
  Mux/1 -> CR CM CN/1
  sin26/1 -> ROLL/17(dsr), PITCH/15(dsr), YAW/14(dsr)

== system gtm_aeromodel/get aero forces and moments/AERODYNAMICS/NONDIMRATE ==
  P Q R : Inport  OutDataType=sfix(16)  OutScaling=2^0
  alpha beta eps_h alpha_h : Inport  Port=2  OutDataType=sfix(16)  OutScaling=2^0
  Vtas EASkts Mach Qdyn CASkts : Inport  Port=3  OutDataType=sfix(16)  OutScaling=2^0
  Demux1 : Demux  Outputs=3
  Fcn : Fcn  Expr=u(1)*u(6)/(2*u(5))
  Fcn2 : Fcn  Expr=u(2)*u(7)/(2*u(5))
  Fcn3 : Fcn  Expr=u[1]
  Fcn4 : Fcn  Expr=u[1]
  Fcn6 : Fcn  Expr=u(3)*u(6)/(2*u(5))
  Gain : Gain  Gain=pi/180  ParameterDataType=sfix(16)  ParameterScaling=2^0  OutDataType=sfix(16)  OutScaling=2^0  SaturateOnIntegerOverflow=on  OutDataTypeStr=Inherit: Same as input  ParamDataTypeStr=Inherit: Same as input
  Mux : Mux  Inputs=7
  Mux5 : Mux  Inputs=3
  R2D1 : Gain  Gain=[1 1 1]  ParameterDataType=sfix(16)  ParameterScaling=2^0  OutDataType=sfix(16)  OutScaling=2^0  SaturateOnIntegerOverflow=on  OutDataTypeStr=Inherit: Same as input  ParamDataTypeStr=Inherit: Same as input
  Ref. wing chord : Constant  Value=A_CW  OutDataType=sfix(16)  OutScaling=2^0
  Ref. wing span : Constant  Value=A_BW  OutDataType=sfix(16)  OutScaling=2^0
  P' Q' R' : Outport  OutDataType=sfix(16)  OutScaling=2^0
  wires:
  Fcn6/1 -> Mux5/3
  Fcn2/1 -> Mux5/2
  Fcn/1 -> Mux5/1
  R2D1/1 -> P' Q' R'/1
  Mux5/1 -> R2D1/1
  Fcn3/1 -> Gain/1
  Gain/1 -> Mux/4
  Mux/1 -> Fcn2/1, Fcn6/1, Fcn/1
  Ref. wing chord/1 -> Mux/7
  Ref. wing span/1 -> Mux/6
  Fcn4/1 -> Mux/5
  Demux1/3 -> Mux/3
  Demux1/2 -> Mux/2
  Demux1/1 -> Mux/1
  Vtas EASkts Mach Qdyn CASkts/1 -> Fcn4/1
  P Q R/1 -> Demux1/1
  alpha beta eps_h alpha_h/1 -> Fcn3/1

== system gtm_aeromodel/get aero forces and moments/AERODYNAMICS/XFORMATION of  AERO FORCES and MOMENTS   to cg centered body axis ==
  note: Cx
      | Cy
      | Cz
  note: CRb
      | CMb
      | CNb
  note: CRcg
      | CMcg
      | CNcg
  Vtas EASkts Mach Qdyn CASkts : Inport  OutDataType=sfix(16)  OutScaling=2^0
  CL CD CY : Inport  Port=2  OutDataType=sfix(16)  OutScaling=2^0
  alpha beta alpha_dot beta_dot : Inport  Port=3  OutDataType=sfix(16)  OutScaling=2^0
  CR CM CN : Inport  Port=4  OutDataType=sfix(16)  OutScaling=2^0
  FScg WLcg BLcg : Inport  Port=5  OutDataType=sfix(16)  OutScaling=2^0
  CP2CG : Subsystem
  DIMENSION : Subsystem
  STAB2BODY : Subsystem
  Xa Ya Za : Outport  OutDataType=sfix(16)  OutScaling=2^0  InitialOutput=0
  La Ma Na : Outport  Port=2  OutDataType=sfix(16)  OutScaling=2^0  InitialOutput=0
  wires:
  STAB2BODY/2(CRb CMb CNb) -> CP2CG/2(CRb CMb CNb)
  CR CM CN/1 -> STAB2BODY/3(CR CM CN)
  CP2CG/1(CRcg CMcg CNcg) -> DIMENSION/3(CRcg CMcg CNcg)
  FScg WLcg BLcg/1 -> CP2CG/3(FScg WLcg BLcg)
  DIMENSION/2(La Ma Na) -> La Ma Na/1
  DIMENSION/1(Xa Ya Za) -> Xa Ya Za/1
  CL CD CY/1 -> STAB2BODY/2(CL CD CY)
  Vtas EASkts Mach Qdyn CASkts/1 -> DIMENSION/1(Vtas EASkts Mach Qdyn CASkts)
  alpha beta alpha_dot beta_dot/1 -> STAB2BODY/1(alpha beta alpha_dot beta_dot)
  STAB2BODY/1(Cx Cy Cz) -> DIMENSION/2(Cx Cy Cz), CP2CG/1(Cx Cy Cz)

== system gtm_aeromodel/get prop forces and moments/ENGINE/EPRn/Tra1 ==
  X : Inport  OutDataType=sfix(16)  OutScaling=2^0
  Y : Inport  Port=2  OutDataType=sfix(16)  OutScaling=2^0
  Z : Inport  Port=3  OutDataType=sfix(16)  OutScaling=2^0
  Mux : Mux  Inputs=3
  S-Function : S-Function  FunctionName=table3v5  Parameters=x,y,z,tab  EnableBusSupport=off
  Interp Value : Outport  OutDataType=sfix(16)  OutScaling=2^0
  wires:
  Z/1 -> Mux/3
  Y/1 -> Mux/2
  X/1 -> Mux/1
  Mux/1 -> S-Function/1
  S-Function/1 -> Interp Value/1

== system gtm_aeromodel/get prop forces and moments/ENGINE/Fnt/EPRn ==
  X : Inport  OutDataType=sfix(16)  OutScaling=2^0
  Y : Inport  Port=2  OutDataType=sfix(16)  OutScaling=2^0
  Z : Inport  Port=3  OutDataType=sfix(16)  OutScaling=2^0
  Mux : Mux  Inputs=3
  S-Function : S-Function  FunctionName=table3v5  Parameters=x,y,z,tab  EnableBusSupport=off
  Interp Value : Outport  OutDataType=sfix(16)  OutScaling=2^0
  wires:
  Z/1 -> Mux/3
  Y/1 -> Mux/2
  X/1 -> Mux/1
  Mux/1 -> S-Function/1
  S-Function/1 -> Interp Value/1

== system gtm_aeromodel/get prop forces and moments/ENGINE/Fnt/EPRn1 ==
  X : Inport  OutDataType=sfix(16)  OutScaling=2^0
  Y : Inport  Port=2  OutDataType=sfix(16)  OutScaling=2^0
  Z : Inport  Port=3  OutDataType=sfix(16)  OutScaling=2^0
  Mux : Mux  Inputs=3
  S-Function : S-Function  FunctionName=table3v5  Parameters=x,y,z,tab  EnableBusSupport=off
  Interp Value : Outport  OutDataType=sfix(16)  OutScaling=2^0
  wires:
  S-Function/1 -> Interp Value/1
  Mux/1 -> S-Function/1
  X/1 -> Mux/1
  Y/1 -> Mux/2
  Z/1 -> Mux/3

== system gtm_aeromodel/get prop forces and moments/ENGINE/Fnt/EPRn2 ==
  X : Inport  OutDataType=sfix(16)  OutScaling=2^0
  Y : Inport  Port=2  OutDataType=sfix(16)  OutScaling=2^0
  Z : Inport  Port=3  OutDataType=sfix(16)  OutScaling=2^0
  Mux : Mux  Inputs=3
  S-Function : S-Function  FunctionName=table3v5  Parameters=x,y,z,tab  EnableBusSupport=off
  Interp Value : Outport  OutDataType=sfix(16)  OutScaling=2^0
  wires:
  Z/1 -> Mux/3
  Y/1 -> Mux/2
  X/1 -> Mux/1
  Mux/1 -> S-Function/1
  S-Function/1 -> Interp Value/1

== system gtm_aeromodel/get prop forces and moments/ENGINE/TRA Normalization1 ==
  note: Model Name: TRA NORMALIZATION    Rev.: -
      | Description: Tra Normalization Diagram
      | PCR: N/A    Next Block: ENGINE PARAMETER COMPUTATIONS
      | Written By: K. GOODWIN    Date: 10-18-99
  Tra : Inport  OutDataType=sfix(16)  OutScaling=2^0
  Constant : Constant  Value=2  OutDataType=sfix(16)  OutScaling=2^0
  Constant1 : Constant  Value=37.5  OutDataType=sfix(16)  OutScaling=2^0
  Product : Product  Inputs=*/  OutDataType=sfix(16)  OutScaling=2^0  SaturateOnIntegerOverflow=on  RndMeth=Zero  InputSameDT=on  OutDataTypeStr=Inherit: Same as first input
  Sum : Sum  Inputs=+-  OutDataType=sfix(16)  OutScaling=2^0  SaturateOnIntegerOverflow=on  InputSameDT=on  OutDataTypeStr=Inherit: Same as first input
  Sum1 : Sum  Inputs=-+  OutDataType=sfix(16)  OutScaling=2^0  SaturateOnIntegerOverflow=on  InputSameDT=on  OutDataTypeStr=Inherit: Same as first input
  Tran : Outport  OutDataType=sfix(16)  OutScaling=2^0
  wires:
  Tra/1 -> Sum/1
  Constant/1 -> Sum/2, Sum1/1
  Constant1/1 -> Sum1/2
  Sum/1 -> Product/1
  Sum1/1 -> Product/2
  Product/1 -> Tran/1

== system gtm_aeromodel/aero surf ganging/SPOILER/Model Info/EmptySubsystem ==

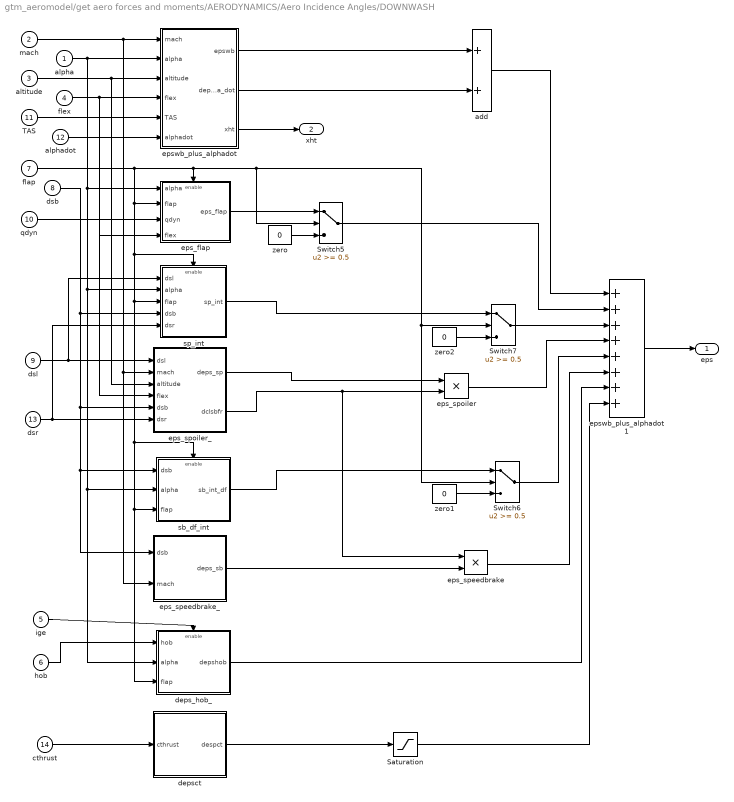
== system gtm_aeromodel/get aero forces and moments/AERODYNAMICS/Aero Incidence Angles/DOWNWASH ==
  "alpha " : Inport  OutDataType=sfix(16)  OutScaling=2^0
  mach : Inport  Port=2  OutDataType=sfix(16)  OutScaling=2^0
  altitude : Inport  Port=3  OutDataType=sfix(16)  OutScaling=2^0
  flex : Inport  Port=4  OutDataType=sfix(16)  OutScaling=2^0
  ige : Inport  Port=5  OutDataType=sfix(16)  OutScaling=2^0
  hob : Inport  Port=6  OutDataType=sfix(16)  OutScaling=2^0
  flap : Inport  Port=7  OutDataType=sfix(16)  OutScaling=2^0
  dsb : Inport  Port=8  OutDataType=sfix(16)  OutScaling=2^0
  dsl : Inport  Port=9  OutDataType=sfix(16)  OutScaling=2^0
  qdyn : Inport  Port=10  OutDataType=sfix(16)  OutScaling=2^0
  TAS : Inport  Port=11  OutDataType=sfix(16)  OutScaling=2^0
  alphadot : Inport  Port=12  OutDataType=sfix(16)  OutScaling=2^0
  dsr : Inport  Port=13  OutDataType=sfix(16)  OutScaling=2^0
  cthrust : Inport  Port=14  OutDataType=sfix(16)  OutScaling=2^0
  Saturation : Saturate  UpperLimit=inf  LowerLimit=-4.5
  Switch5 : Switch  Threshold=0.5  SaturateOnIntegerOverflow=on  InputSameDT=on
  Switch6 : Switch  Threshold=0.5  SaturateOnIntegerOverflow=on  InputSameDT=on
  Switch7 : Switch  Threshold=0.5  SaturateOnIntegerOverflow=on  InputSameDT=on
  add : Sum  OutDataType=sfix(16)  OutScaling=2^0  SaturateOnIntegerOverflow=on  InputSameDT=on  OutDataTypeStr=Inherit: Same as first input
  deps_hob_ : Subsystem  TreatAsAtomicUnit=on
  depsct : Subsystem
  eps_flap : Subsystem  TreatAsAtomicUnit=on
  eps_speedbrake : Product  OutDataType=sfix(16)  OutScaling=2^0  SaturateOnIntegerOverflow=on  RndMeth=Zero  InputSameDT=on  OutDataTypeStr=Inherit: Same as first input
  eps_speedbrake_ : Subsystem
  eps_spoiler : Product  OutDataType=sfix(16)  OutScaling=2^0  SaturateOnIntegerOverflow=on  RndMeth=Zero  InputSameDT=on  OutDataTypeStr=Inherit: Same as first input
  eps_spoiler_ : Subsystem
  epswb_plus_alphadot : Subsystem
  epswb_plus_alphadot 1 : Sum  Inputs=++++++++  OutDataType=sfix(16)  OutScaling=2^0  SaturateOnIntegerOverflow=on  InputSameDT=on  OutDataTypeStr=Inherit: Same as first input
  sb_df_int : Subsystem  TreatAsAtomicUnit=on
  sp_int : Subsystem  TreatAsAtomicUnit=on
  zero : Constant  Value=0  OutDataType=sfix(16)  OutScaling=2^0
  zero1 : Constant  Value=0  OutDataType=sfix(16)  OutScaling=2^0
  zero2 : Constant  Value=0  OutDataType=sfix(16)  OutScaling=2^0
  eps : Outport  OutDataType=sfix(16)  OutScaling=2^0
  xht : Outport  Port=2  OutDataType=sfix(16)  OutScaling=2^0
  wires:
  Saturation/1 -> epswb_plus_alphadot 1/8
  depsct/1(despct) -> Saturation/1
  Switch5/1 -> epswb_plus_alphadot 1/2
  eps_speedbrake/1 -> epswb_plus_alphadot 1/6
  deps_hob_/1(depshob) -> epswb_plus_alphadot 1/7
  Switch6/1 -> epswb_plus_alphadot 1/5
  eps_spoiler/1 -> epswb_plus_alphadot 1/4
  epswb_plus_alphadot 1/1 -> eps/1
  Switch7/1 -> epswb_plus_alphadot 1/3
  epswb_plus_alphadot/2(deps_alpha_dot) -> add/2
  epswb_plus_alphadot/1(epswb) -> add/1
  alphadot/1 -> epswb_plus_alphadot/6(alphadot)
  TAS/1 -> epswb_plus_alphadot/5(TAS)
  add/1 -> epswb_plus_alphadot 1/1
  qdyn/1 -> eps_flap/3(qdyn)
  zero/1 -> Switch5/3
  eps_flap/1(eps_flap) -> Switch5/1
  flap/1 -> sp_int/3(flap), sb_df_int/3(flap), deps_hob_/3(flap), sb_df_int/Enable, sp_int/Enable, eps_flap/2(flap), Switch7/2, Switch6/2, Switch5/2, eps_flap/Enable
  zero2/1 -> Switch7/3
  sp_int/1(sp_int) -> Switch7/1
  "alpha "/1 -> epswb_plus_alphadot/2("alpha "), deps_hob_/2(alpha), sb_df_int/2(alpha), sp_int/2(alpha), eps_flap/1(alpha)
  altitude/1 -> eps_spoiler_/3(altitude), epswb_plus_alphadot/3(altitude)
  flex/1 -> eps_spoiler_/4(flex), eps_flap/4(flex), epswb_plus_alphadot/4(flex)
  mach/1 -> epswb_plus_alphadot/1(mach), eps_spoiler_/2(mach), eps_speedbrake_/2(mach)
  hob/1 -> deps_hob_/1(hob)
  ige/1 -> deps_hob_/Enable
  zero1/1 -> Switch6/3
  dsl/1 -> sp_int/1(dsl), eps_spoiler_/1(dsl)
  eps_spoiler_/2(dclsbfr) -> eps_speedbrake/1, eps_spoiler/2
  eps_spoiler_/1(deps_sp) -> eps_spoiler/1
  cthrust/1 -> depsct/1(cthrust)
  dsb/1 -> sp_int/4(dsb), sb_df_int/1(dsb), eps_speedbrake_/1(dsb), eps_spoiler_/5(dsb)
  sb_df_int/1(sb_int_df) -> Switch6/1
  eps_speedbrake_/1(deps_sb) -> eps_speedbrake/2
  dsr/1 -> eps_spoiler_/6(dsr), sp_int/5(dsr)
  epswb_plus_alphadot/3(xht) -> xht/1
